simulink model "fwv_modified"  (R2021b)
settings: Solver=ode15s  StartTime=0.0  StopTime=10  FixedStep=0.01  MaxStep=0.01  RelTol=1e-3  AbsTol=1e-3  EnableMultiTasking=on
model workspace (MATLAB code in the model file):
  | p0=[0 0 0];
undefined symbols (not defined in the file): A_D, A_L, adpk, adps, c_bar, C_D0, il, ol, psi0, r00, r11, r22, r33, r_cp, rho, Rw, X, Y, Z, z00, z11, z22, zrd
libraries: sm_lib x54, nesl_utility x45, vrlib x3
(part 1 of 3)
settings Model: NumberOfSteps=10  PacingRate=1000  Creator=jeff  LastModifiedBy=jeff
settings SolverCC: AutoScaleAbsTol=off  ZeroCrossAlgorithm=Adaptive  SolverResetMethod=Robust
settings DataIOCC: LimitDataPoints=on  MaxDataPoints=10000  SignalLogging=off  DSMLogging=off  InspectSignalLogs=on  SaveTime=off  ReturnWorkspaceOutputs=off
settings OptimizationCC: LifeSpan=inf
settings DebuggingCC: AllowSymbolicDim=off  SFUnexpectedBacktrackingDiag=warning  SFNoUnconditionalDefaultTransitionDiag=warning  SFExecutionAtInitializationDiag=none  SFMachineParentedDataDiag=warning  ArithmeticOperatorsInVariantConditions=warning
settings ModelReferenceCC: ModelReferenceMinAlgLoopOccurrences=on
settings SFSimCC: SimUseLocalCustomCode=off  CustomCodeUndefinedFunction=UseInterfaceOnly
settings RTWCC: RTWUseLocalCustomCode=off
settings CodeAppCC: StateflowObjectComments=on
settings GRTTargetCC: TargetLangStandard=C89/C90 (ANSI)
settings ConfigComp: CovMetricSettings=dw  CovSaveCumulativeToWorkspaceVar=on  CovSaveSingleToWorkspaceVar=on  CovExternalEMLEnable=off  CovSFcnEnable=off
settings SimscapeCC: SimscapeLogType=all  SimscapeLogSimulationStatistics=on  SimscapeLogDataHistory=10000
settings ExplorerConfigSet: InternalSimMechanicsExplorerSettings="<ExplorerConfiguration><canonicalview>default</canonicalview><AnimationSetting><BasePlaybackSpeed>1.0</BasePlaybackSpeed><PlaybackSpeedFactor>1.0</PlaybackSpeedFactor></AnimationSetting><TilePanel><TileInfo><Tiles Columns=\"2\" Count=\"4\" Rows=\"2\"><Column Weight=\"0.5\"/><Column Weight=\"0.5\"/><Row Weight=\"0.4982\"/><Row Weight=\"0.5018\"/><Tile Height=\"1\" Width=\"1\" X=\"0\" Y=\"0\"/><Tile Height=\"1\" Width=\"1\" X=\"0\" Y=\"1\"/><Tile Height=\"1\" Width=\"1\" X=\"1\" Y=\"0\"/><Tile Height=\"1\" Width=\"1\" X=\"1\" Y=\"1\"/></Tiles></TileInfo><SceneInfo><SceneViewer><BGColor><R>1</R><G>1</G><B>1</B></BGColor><Camera><DoPerspective>off</DoPerspective><Position><X>0.641396731553975696</X><Y>-14.1815569735496414</Y><Z>0.672169191527196008</Z></Position><Center><X>0.641396731553975696</X><Y>-2.76871848114979002e-07</Y><Z>0.672169191527196008</Z></Center><Up><X>0</X><Y>-0</Y><Z>1</Z></Up><ViewLimDist>1</ViewLimDist><YLim>0.799989355072956321</YLim><XLim>1.08260667709303204</XLim></Camera></SceneViewer><SceneViewer><BGColor><R>1</R><G>1</G><B>1</B></BGColor><Camera><DoPerspective>off</DoPerspective><Position><X>-0.159012287126067881</X><Y>0.579024453304961995</Y><Z>14.2124818348279263</Z></Position><Center><X>-0.159012287126067881</X><Y>0.579024453304961995</Y><Z>-0.00300049176476058221</Z></Center><Up><X>0</X><Y>1</Y><Z>-0</Z></Up><ViewLimDist>1</ViewLimDist><YLim>3.05791516459476309</YLim><XLim>4.10313475475286005</XLim></Camera></SceneViewer><SceneViewer><BGColor><R>1</R><G>1</G><B>1</B></BGColor><Camera><DoPerspective>off</DoPerspective><Position><X>14.1815569760706541</X><Y>0.198096922096877126</Y><Z>0.664029497099502652</Z></Position><Center><X>-9.47977211396278108e-07</X><Y>0.198096922096877126</Y><Z>0.664029497099502652</Z></Center><Up><X>-0</X><Y>0</Y><Z>1</Z></Up><ViewLimDist>1</ViewLimDist><YLim>0.784069566907004467</YLim><XLim>1.06106280421888055</XLim></Camera></SceneViewer><SceneViewer><BGColor><R>1</R><G>1</G><B>1</B></BGColor><Camera><DoPerspective>on</DoPerspective><Position><X>0.900649549639901181</X><Y>0.398934934644883776</Y><Z>0.90015424109364861</Z></Position><Center><X>0.500649549639901048</X><Y>0.398934934644883721</Y><Z>0.800154241093648633</Z></Center><Up><X>0</X><Y>-3.08148791101957736e-33</Y><Z>1</Z></Up><ViewLimDist>1</ViewLimDist><YLim>0.466307658154998583</YLim><XLim>0.625695304021537613</XLim></Camera></SceneViewer></SceneInfo></TilePanel><MechEditorPanel><Cameras><Camera><Id>Camera1</Id><Value><Name>Camera1</Name><NativeCamera><PositionTrackingFeature>FWV.Body.camera.camera_Frame.R</PositionTrackingFeature><CenterTrackingFeature>FWV.Body.camera.C</CenterTrackingFeature><UpVectorTrackingFeature>FWV.Body.camera.C</UpVectorTrackingFeature><CenterTrackingOrigin>on</CenterTrackingOrigin><UpVectorTrackingDirection>+Z</UpVectorTrackingDirection></NativeCamera></Value></Camera></Cameras><GfxPanelCameraMap><MapElement CameraMLId=\"Camera1\" GfxPanelIndex=\"3\"/></GfxPanelCameraMap><VideoCreator><PlaybackSpeedRatio>1.0</PlaybackSpeedRatio><FrameRate>30</FrameRate><VideoFormat>Motion JPEG AVI</VideoFormat><FrameSize>[1280 720]</FrameSize></VideoCreator></MechEditorPanel></ExplorerConfiguration>"

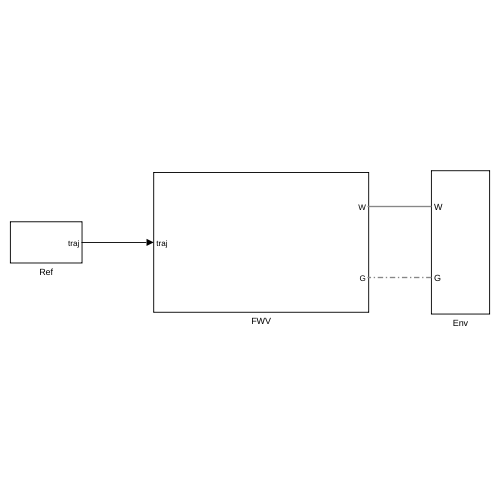
[thumbnail: Simulink's stored preview of the top-level diagram]
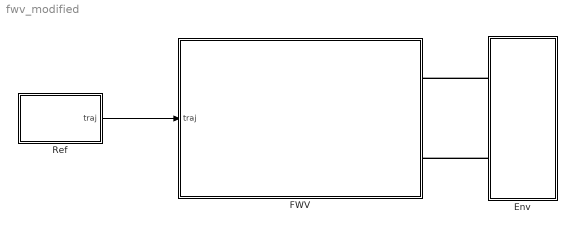
== system fwv_modified ==
  Env : Subsystem
  FWV : Subsystem
  Ref : Subsystem
  wires:
  Ref/1(traj) -> FWV/1(traj)
  connections:
  Env/LConn1 -- FWV/RConn1
  Env/LConn2 -- FWV/RConn2

== system fwv_modified/Env ==
  Ground : Subsystem
  Mechanism Configuration : sm_lib/Utilities/Mechanism Configuration  UniformGravity=Constant  GravityVector=[0 0 -9.80665]  GravityUnits=m/s^2  LinearizationDelta=0.001  JointModeTransitionNonlinearIterations=2
  Solver Configuration : nesl_utility/Solver Configuration  PhysicalDomain=network_engine_domain  SubClassName=solver  LeftPortType=input  RightPortType=generic  Tones=[]  Harmonics=[]  SimulateNoise=off  Profile=off  UseLocalSampling=off  EnableSwitchedLinearOptims=on  FrequencyDomain=off  UseCCode=off  RelTol=0.001  AbsTol=1e-06  MinStep=1e-09  ToWorkspace=off  RevertToSquareIcSolve=off  NumHomotopyIterations=100  PhasorMode=off  PhasorModeNumHarmonics=1  DoDC=off  ResidualTolerance=1e-09  UseLocalSolver=off  LocalSolverChoice=NE_BACKWARD_EULER_ADVANCER  LocalSolverSampleTime=0.001  DoFixedCost=off  MaxNonlinIter=3  MaxModeIter=2  ComputeImpulses=off  ImpulseIterations=2  LinearAlgebra=Sparse  EquationFormulation=NE_TIME_EF  DelaysMemoryBudget=1024  AutomaticFiltering=on  FilteringTimeConstant=0.001  PartitionStorageMethod=AS_NEEDED  PartitionMemoryBudget=1024  PartitionMethod=FAST
      settings: SourceProductBaseCode=PW,SS
  World Frame1 : sm_lib/Frames and Transforms/World Frame
  W : PMIOPort  Side=Left
  G : PMIOPort  Port=2  Side=Left
  connections:
  Ground/RConn1 -- G/RConn1
  Ground/LConn1 -- Mechanism Configuration/RConn1 -- World Frame1/RConn1 -- Solver Configuration/RConn1 -- W/RConn1

== system fwv_modified/FWV ==
  traj : Inport
  Body : Subsystem  mask{rho_w=900, m_t=20, stif_stk=0, stif_rot=5e-2, damp_rot=0, stif_m=1e2, damp_m=1e2, p0=p0, phi0=0, theta0=0, psi0=psi0}
      mask prompts: p0 "initial position(m)"; phi0 "initial roll(rad)"; theta0 "initial pitch(rad)"; psi0 "initial yaw(rad)"
      mask Display: image('Images/fwv.png');
  Controller : Subsystem
  Visualization : Subsystem
  W : PMIOPort  Side=Right
  G : PMIOPort  Port=2  Side=Right
  wires:
  Controller/1(ctrl) -> Body/1(ctrl)
  Body/1(state) -> Visualization/1(state), Controller/1(state)
  traj/1 -> Visualization/2(traj), Controller/2(Traj)
  connections:
  W/RConn1 -- Body/LConn1
  G/RConn1 -- Body/RConn1

== system fwv_modified/Ref ==
  Clock : Clock
  Mux : Mux  Inputs=6
  To Workspace : ToWorkspace  VariableName=t  SampleTime=-1
  p,pdot,pddot : MATLAB Function  TreatAsAtomicUnit=on
  traj : Outport
  wires:
  Mux/1 -> traj/1
  p,pdot,pddot/1(p) -> Mux/1  "p"
  p,pdot,pddot/2(heading) -> Mux/2
  p,pdot,pddot/3(v) -> Mux/3  "v"
  p,pdot,pddot/4(heading_dot) -> Mux/4
  p,pdot,pddot/5(a) -> Mux/5  "a"
  p,pdot,pddot/6(heading_ddot) -> Mux/6
  Clock/1 -> To Workspace/1, p,pdot,pddot/1(t)

== system fwv_modified/Env/Ground ==
  Cylindrical Solid : sm_lib/Body Elements/Cylindrical Solid  GraphicAmbientColor=[0.15 0.15 0.15 1.0]  BasedOnType=Mass  CenterOfMass=[0 0 0]  CenterOfMassUnits=m  GraphicDiffuseColor=[0.8 1.0 0.8]  CylinderLength=10  CylinderLengthUnits=mm  CylinderRadius=4  CylinderRadiusUnits=m  Density=1000  DensityUnits=kg/m^3  DoExposeReferenceFrame=off  GraphicEmissiveColor=[0.0 0.0 0.0 1.0]  ExportEntireGeometry=on  SerializedFrames=<Frames><Frame><Id>Frame1</Id><Value><Name>F1</Name><Origin><Source>GeometricFeature</Source><FeatureName>top surface</FeatureName></Origin><PrimaryAxis><DefinedDirection>+Z</DefinedDirection><Source>ReferenceFrame</Source><SourceDirection>+Z</SourceDirection><FeatureName></FeatureName></PrimaryAxis><SecondaryAxis><DefinedDirection>+X</DefinedDirection><Source>ReferenceFrame</Source><SourceDirection>+X</SourceDirection><FeatureName></FeatureName></SecondaryAxis></Value></Frame></Frames>  MarkerShape=Sphere  MarkerSize=10  GraphicType=FromGeometry  InertiaType=Custom  Mass=0  MassUnits=kg  MomentsOfInertia=[1 1 1]  MomentsOfInertiaUnits=kg*m^2  GraphicOpacity=1.0  ProductsOfInertia=[0 0 0]  ProductsOfInertiaUnits=kg*m^2  GraphicShininess=75  GraphicSpecularColor=[0.5 0.5 0.5 1.0]  GraphicVisPropType=SimpleVisualProperties
  Rigid Transform : sm_lib/Frames and Transforms/Rigid Transform  TranslationMethod=StandardAxis  TranslationStandardOffset=6  TranslationLengthUnit=cm  TranslationStandardAxis=-Z  TranslationCartesianOffset=[0 0 0]  TranslationROffset=0  TranslationROffsetUnits=m  TranslationZOffset=0  TranslationZOffsetUnits=m  TranslationThetaOffset=0  TranslationThetaOffsetUnits=deg  RotationMethod=None  RotationAngleUnits=deg  RotationStandardAxis=+Z  RotationAngle=0.0  RotationArbitraryAxis=[0 0 1]  FollAlignAxisA=+X  BaseAlignAxisA=+Y  FollAlignAxisB=+Y  BaseAlignAxisB=+Z  RotationSequenceAxes=FollowerAxes  RotationSequence=XYX  RotationSequenceAngles=[0 0 0]  RotationSequenceAnglesUnits=deg  RotationMatrix=[1 0 0; 0 1 0; 0 0 1]
  W : PMIOPort  Side=Left
  G : PMIOPort  Port=2  Side=Right
  connections:
  G/RConn1 -- Cylindrical Solid/RConn1
  Rigid Transform/LConn1 -- W/RConn1
  Rigid Transform/RConn1 -- Cylindrical Solid/LConn1

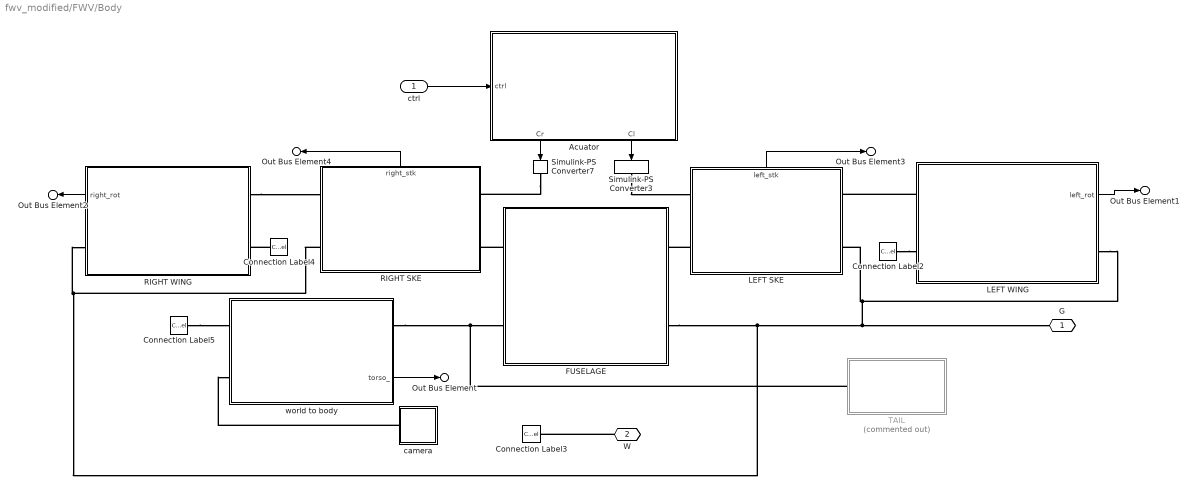
== system fwv_modified/FWV/Body ==
  ctrl : Inport
  Acuator : Subsystem
      settings: PortSchema="{\"entries\":[{\"content\":{\"sides\":[{\"content\":{\"connectorIds\":[\"In1\"]},\"type\":\"ConnectorPlacement.EquallySpacedRectSide\",\"uuid\":\"db46f0ff-2b35-4735-b2ba-99ebad500531\"},{\"content\":{\"connectorIds\":[],\"side\":\"RIGHT\"},\"type\":\"ConnectorPlacement.EquallySpacedRectSide\",\"uuid\":\"a05d2a9d-5b8e-445a-bb52-abca9ea78047\"},{\"content\":{\"connectorIds\":[],\"side\":\"TOP\"},\"type\":\"ConnectorPlacement.EquallySpacedRectSide\",\"uuid\":\"a9e07a0b-59af-45c6-89e8-be07490c71bb\"},{\"content\":{\"connectorIds\":[\"Out1\",\"Out2\"],\"side\":\"BOTTOM\"},\"type\":\"ConnectorPlacement.EquallySpacedRectSide\",\"uuid\":\"69a70806-995a-45b1-874e-667630f2a15c\"}]},\"type\":\"ConnectorPlacement.EquallySpacedConnector\",\"uuid\":\"cc8e5811-56fa-45cd-8c97-474062c30ea3\"}],\"packageUris\":[\"http://schema.mathworks.com/mf0/Connector/R2020b\"],\"version\":\"1.0\"}"
  Connection Label{2..5} (4 alike) : ConnectionLabel  Label=W
  FUSELAGE : Subsystem  mask{mu0=0, mu1=0}
      mask Display: image('Images/fuselage.png'); % Use "Edit Image" on toolstrip to change.
  LEFT SKE : Subsystem
      settings: PortSchema="{\"entries\":[{\"content\":{\"sides\":[{\"content\":{\"connectorIds\":[\"LConn1\",\"LConn2\"]},\"type\":\"ConnectorPlacement.EquallySpacedRectSide\",\"uuid\":\"e449d641-3a3a-4b99-9659-b7cfb3580d3e\"},{\"content\":{\"connectorIds\":[\"RConn1\",\"RConn2\"],\"side\":\"RIGHT\"},\"type\":\"ConnectorPlacement.EquallySpacedRectSide\",\"uuid\":\"c0f0c2d4-a937-4da0-b288-84b9bdeda0ec\"},{\"content\":{\"connectorIds\":[\"Out1\"],\"side\":\"TOP\"},\"type\":\"ConnectorPlacement.EquallySpacedRectSide\",\"uuid\":\"2e9a5fca-fc91-474a-9824-391ef1d64046\"}]},\"type\":\"ConnectorPlacement.EquallySpacedConnector\",\"uuid\":\"1b8d15a7-e855-4706-95be-75cb969fd455\"}],\"packageUris\":[\"http://schema.mathworks.com/mf0/Connector/R2020b\"],\"version\":\"1.0\"}"
      mask Display: image('Images/lle.png'); % Use "Edit Image" on toolstrip to change.
  LEFT WING : Subsystem
      mask Display: image('Images/lwing.png'); % Use "Edit Image" on toolstrip to change.
  RIGHT SKE : Subsystem
      settings: PortSchema="{\"entries\":[{\"content\":{\"sides\":[{\"content\":{\"connectorIds\":[\"LConn1\",\"LConn2\"]},\"type\":\"ConnectorPlacement.EquallySpacedRectSide\",\"uuid\":\"e80f0529-82a8-4e91-8f70-1f5fff48efb0\"},{\"content\":{\"connectorIds\":[\"RConn1\",\"RConn2\"],\"side\":\"RIGHT\"},\"type\":\"ConnectorPlacement.EquallySpacedRectSide\",\"uuid\":\"c7e3ee7d-7bee-46da-b210-768e5832b89d\"},{\"content\":{\"connectorIds\":[\"Out1\"],\"side\":\"TOP\"},\"type\":\"ConnectorPlacement.EquallySpacedRectSide\",\"uuid\":\"680cbd67-40e5-4a58-a196-f2062cf587c7\"}]},\"type\":\"ConnectorPlacement.EquallySpacedConnector\",\"uuid\":\"7cb1a5ec-7352-40bf-9e6c-a29cba360f94\"}],\"packageUris\":[\"http://schema.mathworks.com/mf0/Connector/R2020b\"],\"version\":\"1.0\"}"
      mask Display: image('Images/rle.png'); % Use "Edit Image" on toolstrip to change.
  RIGHT WING : Subsystem
      mask Display: image('Images/rwing.png'); % Use "Edit Image" on toolstrip to change.
  Simulink-PS Converter3 : nesl_utility/Simulink-PS Converter  PhysicalDomain=network_engine_domain  SubClassName=ps_input  LeftPortType=input  RightPortType=output  PseudoPeriodic=off  Frequencies=[]  NoiseDistribution=none  NoiseParameters=[]  Unit=1  AffineConversion=off  FilteringAndDerivatives=filter  SimscapeFilterOrder=2  InputFilterTimeConstant=0.001  UdotUserProvided=2
      settings: SourceProductBaseCode=PW,SS
  Simulink-PS Converter7 : nesl_utility/Simulink-PS Converter  PhysicalDomain=network_engine_domain  SubClassName=ps_input  LeftPortType=input  RightPortType=output  PseudoPeriodic=off  Frequencies=[]  NoiseDistribution=none  NoiseParameters=[]  Unit=1  AffineConversion=off  FilteringAndDerivatives=filter  SimscapeFilterOrder=2  InputFilterTimeConstant=0.001  UdotUserProvided=0
      settings: SourceProductBaseCode=PW,SS
  TAIL : Subsystem  Commented=on
  camera : Subsystem
  world to body : Subsystem
      settings: PortSchema="{\"entries\":[{\"content\":{\"sides\":[{\"content\":{\"connectorIds\":[\"LConn1\",\"LConn2\"]},\"type\":\"ConnectorPlacement.EquallySpacedRectSide\",\"uuid\":\"67e08b7d-27a7-478e-aa2b-0a29cfb8c4ba\"},{\"content\":{\"connectorIds\":[\"RConn1\",\"Out1\"],\"side\":\"RIGHT\"},\"type\":\"ConnectorPlacement.EquallySpacedRectSide\",\"uuid\":\"af848fd7-c404-4734-a34f-7cffff1411b1\"},{\"content\":{\"connectorIds\":[],\"side\":\"TOP\"},\"type\":\"ConnectorPlacement.EquallySpacedRectSide\",\"uuid\":\"40c86437-2469-4d2e-8b61-7b3eee85e893\"}]},\"type\":\"ConnectorPlacement.EquallySpacedConnector\",\"uuid\":\"cd10b607-3f85-4cd2-a6c3-0d07bf2597bd\"}],\"packageUris\":[\"http://schema.mathworks.com/mf0/Connector/R2020b\"],\"version\":\"1.0\"}"
  G : PMIOPort  Side=Right
  W : PMIOPort  Port=2  Side=Left
  Out Bus Element : Outport  PortName=state  Element=pose
  Out Bus Element3 : Outport  PortName=state  Element=left_stk
  Out Bus Element1 : Outport  PortName=state  Element=left_rot
  Out Bus Element4 : Outport  PortName=state  Element=right_stk
  Out Bus Element2 : Outport  PortName=state  Element=right_rot
  wires:
  LEFT WING/1(left_rot) -> Out Bus Element1/1
  RIGHT WING/1(right_rot) -> Out Bus Element2/1
  world to body/1(torso_) -> Out Bus Element/1
  Acuator/2(Cl) -> Simulink-PS Converter3/1
  Acuator/1(Cr) -> Simulink-PS Converter7/1
  ctrl/1 -> Acuator/1(ctrl)
  LEFT SKE/1(left_stk) -> Out Bus Element3/1
  RIGHT SKE/1(right_stk) -> Out Bus Element4/1
  connections:
  LEFT SKE/LConn2 -- FUSELAGE/RConn1
  FUSELAGE/LConn1 -- RIGHT SKE/RConn2
  Simulink-PS Converter7/RConn1 -- RIGHT SKE/RConn1
  world to body/RConn1 -- TAIL/LConn1 -- FUSELAGE/LConn2
  camera/LConn1 -- world to body/LConn2
  Simulink-PS Converter3/RConn1 -- LEFT SKE/LConn1
  LEFT WING/LConn1 -- LEFT SKE/RConn1
  RIGHT WING/LConn1 -- RIGHT SKE/LConn1
  Connection Label2/LConn1 -- LEFT WING/LConn2
  Connection Label4/LConn1 -- RIGHT WING/LConn2
  Connection Label5/LConn1 -- world to body/LConn1
  W/RConn1 -- Connection Label3/LConn1
  RIGHT SKE/LConn2 -- G/RConn1 -- LEFT SKE/RConn2 -- LEFT WING/RConn1 -- FUSELAGE/RConn2 -- RIGHT WING/RConn1

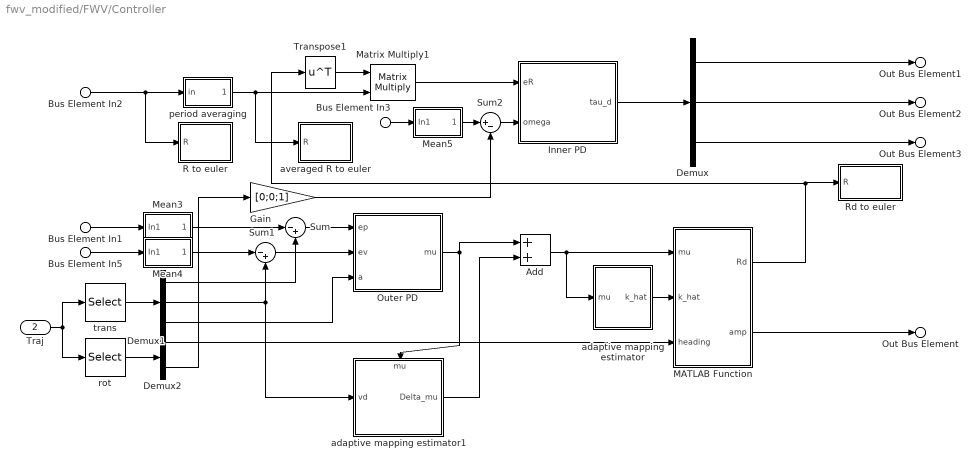
== system fwv_modified/FWV/Controller ==
  Bus Element In1 : Inport  PortName=state  Element=pose.p
  Bus Element In2 : Inport  PortName=state  Element=pose.R
  Bus Element In3 : Inport  PortName=state  Element=pose.w
  Bus Element In5 : Inport  PortName=state  Element=pose.v
  Traj : Inport  Port=2
  Add : Sum
  Demux : Demux  Outputs=3
  Demux1 : Demux  Outputs=3
  Demux2 : Demux  Outputs=2
  Gain : Gain  Gain=[0;0;1]
  Inner PD : Subsystem
  MATLAB Function : MATLAB Function  TreatAsAtomicUnit=on
  Matrix Multiply1 : Product  Multiplication=Matrix(*)
  Mean3 : Subsystem
  Mean4 : Subsystem
  Mean5 : Subsystem
  Outer PD : Subsystem
  R to euler : Subsystem
  Rd to euler : Subsystem
      settings: PortSchema="{\"entries\":[{\"content\":{\"sides\":[{\"content\":{\"connectorIds\":[]},\"type\":\"ConnectorPlacement.EquallySpacedRectSide\",\"uuid\":\"93de112d-0217-40d7-a336-17ea7cc4ed84\"},{\"content\":{\"connectorIds\":[\"In1\"],\"side\":\"RIGHT\"},\"type\":\"ConnectorPlacement.EquallySpacedRectSide\",\"uuid\":\"0b203bc8-f5c1-4f94-b862-0e0b0c3261f7\"},{\"content\":{\"connectorIds\":[],\"side\":\"TOP\"},\"type\":\"ConnectorPlacement.EquallySpacedRectSide\",\"uuid\":\"1be19d4c-6517-470f-aabd-96bb4bcaed3d\"}]},\"type\":\"ConnectorPlacement.EquallySpacedConnector\",\"uuid\":\"f5fc68b0-193c-43e6-a8c2-776496b24de9\"}],\"packageUris\":[\"http://schema.mathworks.com/mf0/Connector/R2020b\"],\"version\":\"1.0\"}"
  Sum : Sum  Inputs=|-+
  Sum1 : Sum  Inputs=|-+
  Sum2 : Sum  Inputs=|+-
  Transpose1 : Math  Operator=transpose  SaturateOnIntegerOverflow=on
  adaptive mapping estimator : Subsystem
  adaptive mapping estimator1 : Subsystem
      settings: PortSchema="{\"entries\":[{\"content\":{\"sides\":[{\"content\":{\"connectorIds\":[\"In1\"]},\"type\":\"ConnectorPlacement.EquallySpacedRectSide\",\"uuid\":\"ad990f9c-fb26-46a0-b20f-9b75f9cabb9c\"},{\"content\":{\"connectorIds\":[\"Out1\"],\"side\":\"RIGHT\"},\"type\":\"ConnectorPlacement.EquallySpacedRectSide\",\"uuid\":\"f73f0012-14a6-4c3b-b3ee-1c6141b5dee9\"},{\"content\":{\"connectorIds\":[\"In2\"],\"side\":\"TOP\"},\"type\":\"ConnectorPlacement.EquallySpacedRectSide\",\"uuid\":\"988c0ea2-b49a-4053-a70e-8b43fa663825\"}]},\"type\":\"ConnectorPlacement.EquallySpacedConnector\",\"uuid\":\"beeb5652-2bef-4034-a2ae-37ff7c082bb3\"}],\"packageUris\":[\"http://schema.mathworks.com/mf0/Connector/R2020b\"],\"version\":\"1.0\"}"
  averaged R to euler : Subsystem
  period averaging : Subsystem
  rot : Selector  InputPortWidth=12  IndexOptions=Index vector (dialog)  Indices=[4 8]  OutputSizes=1
  trans : Selector  InputPortWidth=12  IndexOptions=Index vector (dialog)  Indices=[1 2 3 5 6 7 9 10 11]  OutputSizes=1
  Out Bus Element : Outport  PortName=ctrl  Element=amp_mean
  Out Bus Element1 : Outport  PortName=ctrl  Element=amp_diff
  Out Bus Element2 : Outport  PortName=ctrl  Element=bias
  Out Bus Element3 : Outport  PortName=ctrl  Element=offset
  wires:
  Demux1/1 -> Sum/2
  Inner PD/1(tau_d) -> Demux/1
  Transpose1/1 -> Matrix Multiply1/1
  Demux1/2 -> adaptive mapping estimator1/1(vd), Sum1/2
  Demux1/3 -> Outer PD/3(a)
  Bus Element In2/1 -> R to euler/1(R), period averaging/1(in)
  Demux2/1 -> MATLAB Function/3(heading)
  Sum/1 -> Outer PD/1(ep)
  Sum1/1 -> Outer PD/2(ev)
  Matrix Multiply1/1 -> Inner PD/1(eR)
  MATLAB Function/1(Rd) -> Transpose1/1, Rd to euler/1(R)
  Bus Element In1/1 -> Mean3/1(In1)
  Bus Element In5/1 -> Mean4/1(In1)
  Mean3/1(Mean1) -> Sum/1
  Mean4/1(Mean1) -> Sum1/1
  Bus Element In3/1 -> Mean5/1(In1)
  MATLAB Function/2(amp) -> Out Bus Element/1
  period averaging/1(Mean1) -> averaged R to euler/1(R), Matrix Multiply1/2
  adaptive mapping estimator/1(k_hat) -> MATLAB Function/2(k_hat)
  Demux/1 -> Out Bus Element1/1
  Demux/2 -> Out Bus Element2/1
  Demux/3 -> Out Bus Element3/1
  Mean5/1(Mean1) -> Sum2/1
  Sum2/1 -> Inner PD/2(omega)
  Demux2/2 -> Gain/1
  Gain/1 -> Sum2/2
  trans/1 -> Demux1/1
  rot/1 -> Demux2/1
  Traj/1 -> rot/1, trans/1
  adaptive mapping estimator1/1(Delta_mu) -> Add/2
  Add/1 -> adaptive mapping estimator/1(mu), MATLAB Function/1(mu)
  Outer PD/1(mu) -> adaptive mapping estimator1/2(mu), Add/1

== system fwv_modified/FWV/Visualization ==
  Bus Element In1 : Inport  PortName=state  Element=pose.p
  Bus Element In2 : Inport  PortName=state  Element=pose.R
  traj : Inport  Port=2
  Demux : Demux  Outputs=3
  Mux : Mux  Inputs=2
  Selector : Selector  InputPortWidth=12  IndexOptions=Index vector (dialog)  Indices=[1 2 3 4]  OutputSizes=1
  Subsystem : Subsystem
  Terminator : Terminator
  To Workspace : ToWorkspace  VariableName=q  SampleTime=-1
      settings: Save2DSignal=2-D array (concatenate along first dimension)
  To Workspace1 : ToWorkspace  VariableName=qd  SampleTime=-1
      settings: Save2DSignal=2-D array (concatenate along first dimension)
  XY Graph : Record  FileSettingsInternal="{\"entries\":[{\"content\":{\"excelSettings\":{\"content\":{},\"type\":\"Streamout.ExcelSettings\"}},\"type\":\"Streamout.FileSettingStorage\",\"uuid\":\"9068cc09-93f0-4c38-80ae-0346da1374ca\"}],\"packageUris\":[\"http://schema.mathworks.com/mf0/streamout_blocks/R2020a\"],\"version\":\"1.0\"}"  Layout=[1 1]  SignalsInternal="{\"entries\":[{\"content\":{\"signals\":[{\"content\":{\"blockPath\":[\"fwv_modified/FWV/Visualization/XY Graph\"],\"channel\":[],\"dimensions\":[1],\"domain\":\"fwv_modified/FWV/Visualization/XY Graph\",\"lineColor\":\"#139fff\",\"plots\":[],\"port\":1,\"sid\":[],\"signalID\":199,\"signalName\":\"Demux:1\"},\"type\":\"RecordBlkView.Signal\",\"uuid\":\"b9a14841-9106-4e77-be14-2ac67169168d\"},{\"content\":{\"blockPath\":[\"fwv_modified/FWV/Visualization/XY Graph\"],\"channel\":[],\"dimensions\":[1],\"domain\":\"fwv_modified/FWV/Visualization/XY Graph\",\"lineColor\":\"#ff6929\",\"plots\":[],\"port\":2,\"sid\":[],\"signalID\":202,\"signalName\":\"Demux:2\"},\"type\":\"RecordBlkView.Signal\",\"uuid\":\"9ba150dd-5ced-4f31-a10c-923c26d79fdc\"}]},\"type\":\"RecordBlkView.InputSignals\",\"uuid\":\"991fd4fc-8561-4340-9e61-2b96f507fad7\"}],\"packageUris\":[\"http://schema.mathworks.com/mf0/streamout_blocks/R2020a\"],\"version\":\"1.0\"}"  VisualizationBindings="{\"xyplotplugin\":{\"info\":[{\"series\":[],\"subplotID\":1}]}}"  CompatibilityTag=XY  st=-1
  wires:
  Bus Element In1/1 -> Mux/1, Demux/1
  Demux/3 -> Terminator/1
  Demux/1 -> XY Graph/1
  Demux/2 -> XY Graph/2
  Selector/1 -> To Workspace1/1
  traj/1 -> Selector/1
  Bus Element In2/1 -> Subsystem/1(R)
  Subsystem/1(yaw) -> Mux/2
  Mux/1 -> To Workspace/1

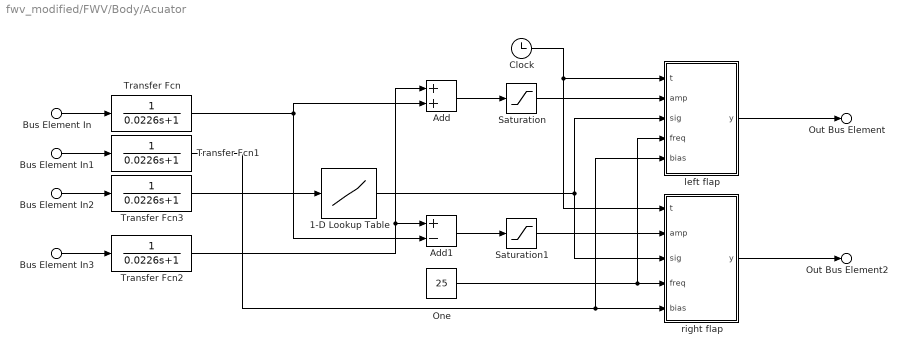
== system fwv_modified/FWV/Body/Acuator ==
  Bus Element In3 : Inport  PortName=ctrl  Element=amp_mean
  Bus Element In : Inport  PortName=ctrl  Element=amp_diff
  Bus Element In1 : Inport  PortName=ctrl  Element=bias
  Bus Element In2 : Inport  PortName=ctrl  Element=offset
  " left flap" : MATLAB Function  TreatAsAtomicUnit=on
  " right flap" : MATLAB Function  TreatAsAtomicUnit=on
  1-D Lookup Table : Lookup_n-D  NumberOfTableDimensions=1  BreakpointsForDimension1=[-1:1]  Table=1.0./(1+exp(-10*[-1:1]))  InternalRulePriority=Speed  RndMeth=Simplest  InputSameDT=on
  Add : Sum
  Add1 : Sum  Inputs=+-
  Clock : Clock
  One : Constant  Value=25  OutDataTypeStr=Inherit: Inherit via back propagation
  Saturation : Saturate  UpperLimit=pi/2  LowerLimit=0  ZeroCross=off
  Saturation1 : Saturate  UpperLimit=pi/2  LowerLimit=0  ZeroCross=off
  Transfer Fcn{,1..3} (4 alike) : TransferFcn  Denominator=[0.0226 1]
  Out Bus Element2 : Outport  PortName=Cr  Element=stroke
  Out Bus Element : Outport  Port=2  PortName=Cl  Element=stroke
  wires:
  Add1/1 -> Saturation1/1
  " left flap"/1(y) -> Out Bus Element/1
  One/1 -> " left flap"/4(freq), " right flap"/4(freq)
  " right flap"/1(y) -> Out Bus Element2/1
  Add/1 -> Saturation/1
  Saturation/1 -> " left flap"/2(amp)
  Clock/1 -> " right flap"/1(t), " left flap"/1(t)
  Saturation1/1 -> " right flap"/2(amp)
  Transfer Fcn2/1 -> Add/1, Add1/1
  Transfer Fcn/1 -> Add1/2, Add/2
  Bus Element In/1 -> Transfer Fcn/1
  Bus Element In1/1 -> Transfer Fcn1/1
  Bus Element In2/1 -> Transfer Fcn3/1
  Bus Element In3/1 -> Transfer Fcn2/1
  Transfer Fcn1/1 -> " left flap"/5(bias), " right flap"/5(bias)
  Transfer Fcn3/1 -> 1-D Lookup Table/1
  1-D Lookup Table/1 -> " right flap"/3(sig), " left flap"/3(sig)

== system fwv_modified/FWV/Body/FUSELAGE ==
  note: Contact Measurement
  Rigid Transform : sm_lib/Frames and Transforms/Rigid Transform  TranslationMethod=StandardAxis  TranslationStandardOffset=5.75  TranslationLengthUnit=cm  TranslationStandardAxis=-Z  TranslationCartesianOffset=[0 0 0]  TranslationROffset=0  TranslationROffsetUnits=m  TranslationZOffset=0  TranslationZOffsetUnits=m  TranslationThetaOffset=0  TranslationThetaOffsetUnits=deg  RotationMethod=RotationSequence  RotationAngleUnits=deg  RotationStandardAxis=+Y  RotationAngle=90  RotationArbitraryAxis=[0 0 1]  FollAlignAxisA=+X  BaseAlignAxisA=+Y  FollAlignAxisB=+Y  BaseAlignAxisB=+Z  RotationSequenceAxes=FollowerAxes  RotationSequence=ZYX  RotationSequenceAngles=[45 90 0]  RotationSequenceAnglesUnits=deg  RotationMatrix=[1 0 0; 0 1 0; 0 0 1]
  Rigid Transform1 : sm_lib/Frames and Transforms/Rigid Transform  TranslationMethod=StandardAxis  TranslationStandardOffset=5.75  TranslationLengthUnit=cm  TranslationStandardAxis=-Z  TranslationCartesianOffset=[0 0 0]  TranslationROffset=0  TranslationROffsetUnits=m  TranslationZOffset=0  TranslationZOffsetUnits=m  TranslationThetaOffset=0  TranslationThetaOffsetUnits=deg  RotationMethod=RotationSequence  RotationAngleUnits=deg  RotationStandardAxis=+X  RotationAngle=90  RotationArbitraryAxis=[0 0 1]  FollAlignAxisA=+X  BaseAlignAxisA=+Y  FollAlignAxisB=+Y  BaseAlignAxisB=+Z  RotationSequenceAxes=FollowerAxes  RotationSequence=ZYX  RotationSequenceAngles=[-45 90 0]  RotationSequenceAnglesUnits=deg  RotationMatrix=[1 0 0; 0 1 0; 0 0 1]
  Spatial Contact Force : sm_lib/Forces and Torques/Spatial Contact Force  CoefficientOfDynamicFriction=0.3  CoefficientOfStaticFriction=0.5  SenseContactBaseRotation=off  SenseContactBaseTranslation=off  NormalDamping=1e3  NormalDampingUnits=N/(m/s)  SenseContactFollowerRotation=off  SenseContactFollowerTranslation=off  SenseContactSignal=off  NormalStiffness=1e6  NormalStiffnessUnits=N/m  FrictionalCriticalVelocity=1e-3  FrictionalCriticalVelocityUnits=m/s  ZeroCrossDetectContactStartAndEnd=off  FrictionType=SmoothStickSlip  SenseFrictionalForceMagnitude=off  SenseNormalForceMagnitude=off  NormalForceType=SmoothSpringDamper  SenseNormalVelocity=off  SenseSeparationDistance=off  SenseTangentialVelocity=off  SenseTangentialVelocityMagnitude=off  NormalTransitionRegionWidth=1e-4  NormalTransitionRegionWidthUnits=m
  Spatial Contact Force1 : sm_lib/Forces and Torques/Spatial Contact Force  CoefficientOfDynamicFriction=0.3  CoefficientOfStaticFriction=0.5  SenseContactBaseRotation=off  SenseContactBaseTranslation=off  NormalDamping=1e3  NormalDampingUnits=N/(m/s)  SenseContactFollowerRotation=off  SenseContactFollowerTranslation=off  SenseContactSignal=off  NormalStiffness=1e6  NormalStiffnessUnits=N/m  FrictionalCriticalVelocity=1e-3  FrictionalCriticalVelocityUnits=m/s  ZeroCrossDetectContactStartAndEnd=off  FrictionType=SmoothStickSlip  SenseFrictionalForceMagnitude=off  SenseNormalForceMagnitude=off  NormalForceType=SmoothSpringDamper  SenseNormalVelocity=off  SenseSeparationDistance=off  SenseTangentialVelocity=off  SenseTangentialVelocityMagnitude=off  NormalTransitionRegionWidth=1e-4  NormalTransitionRegionWidthUnits=m
  Spatial Contact Force2 : sm_lib/Forces and Torques/Spatial Contact Force  CoefficientOfDynamicFriction=0.3  CoefficientOfStaticFriction=0.5  SenseContactBaseRotation=off  SenseContactBaseTranslation=off  NormalDamping=1e3  NormalDampingUnits=N/(m/s)  SenseContactFollowerRotation=off  SenseContactFollowerTranslation=off  SenseContactSignal=off  NormalStiffness=1e6  NormalStiffnessUnits=N/m  FrictionalCriticalVelocity=1e-3  FrictionalCriticalVelocityUnits=m/s  ZeroCrossDetectContactStartAndEnd=off  FrictionType=SmoothStickSlip  SenseFrictionalForceMagnitude=off  SenseNormalForceMagnitude=off  NormalForceType=SmoothSpringDamper  SenseNormalVelocity=off  SenseSeparationDistance=off  SenseTangentialVelocity=off  SenseTangentialVelocityMagnitude=off  NormalTransitionRegionWidth=1e-4  NormalTransitionRegionWidthUnits=m
  left_edge_of_torso : sm_lib/Frames and Transforms/Rigid Transform  TranslationMethod=Cartesian  TranslationStandardOffset=0  TranslationLengthUnit=cm  TranslationStandardAxis=+Z  TranslationCartesianOffset=[0 3.5 0]  TranslationROffset=0  TranslationROffsetUnits=m  TranslationZOffset=0  TranslationZOffsetUnits=m  TranslationThetaOffset=0  TranslationThetaOffsetUnits=deg  RotationMethod=None  RotationAngleUnits=deg  RotationStandardAxis=+Z  RotationAngle=0.0  RotationArbitraryAxis=[0 0 1]  FollAlignAxisA=+X  BaseAlignAxisA=+Y  FollAlignAxisB=+Y  BaseAlignAxisB=+Z  RotationSequenceAxes=FollowerAxes  RotationSequence=XYX  RotationSequenceAngles=[0 0 0]  RotationSequenceAnglesUnits=deg  RotationMatrix=[1 0 0; 0 1 0; 0 0 1]
  leg : sm_lib/Body Elements/Cylindrical Solid  GraphicAmbientColor=[0.15 0.15 0.15 1.0]  BasedOnType=Mass  CenterOfMass=[0 0 0]  CenterOfMassUnits=m  GraphicDiffuseColor=[0.5 0.5 0.5]  CylinderLength=160  CylinderLengthUnits=mm  CylinderRadius=2.5  CylinderRadiusUnits=mm  Density=1000  DensityUnits=kg/m^3  DoExposeReferenceFrame=on  GraphicEmissiveColor=[0.0 0.0 0.0 1.0]  ExportEntireGeometry=on  SerializedFrames=<Frames/>  MarkerShape=Sphere  MarkerSize=10  GraphicType=FromGeometry  InertiaType=CalculateFromGeometry  Mass=1  MassUnits=g  MomentsOfInertia=[1 1 1]  MomentsOfInertiaUnits=kg*m^2  GraphicOpacity=1.0  ProductsOfInertia=[0 0 0]  ProductsOfInertiaUnits=kg*m^2  GraphicShininess=75  GraphicSpecularColor=[0.5 0.5 0.5 1.0]  GraphicVisPropType=SimpleVisualProperties
  leg1 : sm_lib/Body Elements/Cylindrical Solid  GraphicAmbientColor=[0.15 0.15 0.15 1.0]  BasedOnType=Mass  CenterOfMass=[0 0 0]  CenterOfMassUnits=m  GraphicDiffuseColor=[0.5 0.5 0.5]  CylinderLength=160  CylinderLengthUnits=mm  CylinderRadius=2.5  CylinderRadiusUnits=mm  Density=800  DensityUnits=kg/m^3  DoExposeReferenceFrame=on  GraphicEmissiveColor=[0.0 0.0 0.0 1.0]  ExportEntireGeometry=on  SerializedFrames=<Frames/>  MarkerShape=Sphere  MarkerSize=10  GraphicType=FromGeometry  InertiaType=CalculateFromGeometry  Mass=1  MassUnits=g  MomentsOfInertia=[1 1 1]  MomentsOfInertiaUnits=kg*m^2  GraphicOpacity=1.0  ProductsOfInertia=[0 0 0]  ProductsOfInertiaUnits=kg*m^2  GraphicShininess=75  GraphicSpecularColor=[0.5 0.5 0.5 1.0]  GraphicVisPropType=SimpleVisualProperties
  right_edge_of_torso : sm_lib/Frames and Transforms/Rigid Transform  TranslationMethod=Cartesian  TranslationStandardOffset=0  TranslationLengthUnit=cm  TranslationStandardAxis=+Z  TranslationCartesianOffset=[0 -3.5 0]  TranslationROffset=0  TranslationROffsetUnits=m  TranslationZOffset=0  TranslationZOffsetUnits=m  TranslationThetaOffset=0  TranslationThetaOffsetUnits=deg  RotationMethod=StandardAxis  RotationAngleUnits=deg  RotationStandardAxis=+X  RotationAngle=180  RotationArbitraryAxis=[0 0 1]  FollAlignAxisA=+X  BaseAlignAxisA=+Y  FollAlignAxisB=+Y  BaseAlignAxisB=+Z  RotationSequenceAxes=FollowerAxes  RotationSequence=XYX  RotationSequenceAngles=[0 0 0]  RotationSequenceAnglesUnits=deg  RotationMatrix=[1 0 0; 0 1 0; 0 0 1]
  torso : sm_lib/Body Elements/File Solid  ExtGeomFileName=meshes/fuselage.stl  UnitType=Custom  ExtGeomFileUnits=mm  StepReaderType=HEX  ExportConvexHullGeometry=on  InertiaType=CalculateFromGeometry  Mass=m_t  MassUnits=g  CenterOfMass=[0 0 0]  CenterOfMassUnits=cm  MomentsOfInertia=[4e-5, 3e-5, 1.2e-5]  MomentsOfInertiaUnits=kg*m^2  ProductsOfInertia=[0 0 0]  ProductsOfInertiaUnits=kg*m^2  BasedOnType=Mass  Density=1000  DensityUnits=kg/m^3  DoExposeReferenceFrame=on  SerializedFrames=<Frames/>  GraphicType=FromGeometry  MarkerShape=Sphere  MarkerSize=10  GraphicVisPropType=SimpleVisualProperties  GraphicDiffuseColor=[0.5 0.5 0.5]  GraphicSpecularColor=[0.5 0.5 0.5 1.0]  GraphicAmbientColor=[0.15 0.15 0.15 1.0]  GraphicEmissiveColor=[0.0 0.0 0.0 1.0]  GraphicShininess=75  GraphicOpacity=1.0
  F1 : PMIOPort  Side=Right
  F2 : PMIOPort  Port=2  Side=Left
  TS : PMIOPort  Port=3  Side=Left
  G : PMIOPort  Port=4  Side=Right
  connections:
  Spatial Contact Force/RConn1 -- leg/LConn1
  Rigid Transform1/LConn1 -- torso/RConn1 -- right_edge_of_torso/LConn1 -- left_edge_of_torso/LConn1 -- Rigid Transform/LConn1 -- TS/RConn1
  Rigid Transform1/RConn1 -- leg1/RConn1
  left_edge_of_torso/RConn1 -- F1/RConn1
  leg/RConn1 -- Rigid Transform/RConn1
  F2/RConn1 -- right_edge_of_torso/RConn1
  Spatial Contact Force1/RConn1 -- leg1/LConn1
  G/RConn1 -- Spatial Contact Force2/LConn1 -- Spatial Contact Force1/LConn1 -- Spatial Contact Force/LConn1
  Spatial Contact Force2/RConn1 -- torso/LConn1

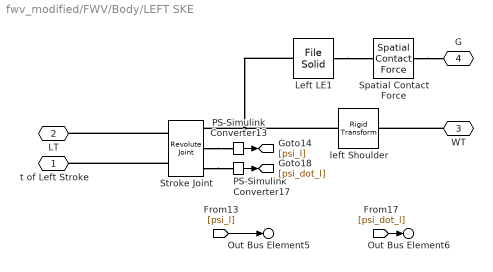
== system fwv_modified/FWV/Body/LEFT SKE ==
  Left LE1 : sm_lib/Body Elements/File Solid  ExtGeomFileName=meshes/left_LE.step  UnitType=FromFile  ExtGeomFileUnits=m  StepReaderType=HEX  ExportConvexHullGeometry=on  InertiaType=Custom  Mass=1  MassUnits=g  CenterOfMass=[0 0.0453 0.0239]  CenterOfMassUnits=m  MomentsOfInertia=[3.2e-06, 7.22e-07, 2.48e-06]  MomentsOfInertiaUnits=kg*m^2  ProductsOfInertia=[-7.2975e-07 0 0]  ProductsOfInertiaUnits=kg*m^2  BasedOnType=Mass  Density=800  DensityUnits=kg/m^3  DoExposeReferenceFrame=on  SerializedFrames=<Frames/>  GraphicType=FromGeometry  MarkerShape=Sphere  MarkerSize=10  GraphicVisPropType=SimpleVisualProperties  GraphicDiffuseColor=[0.5 0.5 0.5]  GraphicSpecularColor=[0.5 0.5 0.5 1.0]  GraphicAmbientColor=[0.15 0.15 0.15 1.0]  GraphicEmissiveColor=[0.0 0.0 0.0 1.0]  GraphicShininess=75  GraphicOpacity=1.0
  PS-Simulink Converter13 : nesl_utility/PS-Simulink Converter  PhysicalDomain=network_engine_domain  SubClassName=ps_output  LeftPortType=input  RightPortType=output  PseudoPeriodic=off  Frequencies=[]  Unit=inherit  AffineConversion=off
      settings: SourceProductBaseCode=PW,SS
  PS-Simulink Converter17 : nesl_utility/PS-Simulink Converter  PhysicalDomain=network_engine_domain  SubClassName=ps_output  LeftPortType=input  RightPortType=output  PseudoPeriodic=off  Frequencies=[]  Unit=inherit  AffineConversion=off
      settings: SourceProductBaseCode=PW,SS
  Spatial Contact Force : sm_lib/Forces and Torques/Spatial Contact Force  CoefficientOfDynamicFriction=0.3  CoefficientOfStaticFriction=0.5  SenseContactBaseRotation=off  SenseContactBaseTranslation=off  NormalDamping=1e3  NormalDampingUnits=N/(m/s)  SenseContactFollowerRotation=off  SenseContactFollowerTranslation=off  SenseContactSignal=off  NormalStiffness=1e6  NormalStiffnessUnits=N/m  FrictionalCriticalVelocity=1e-3  FrictionalCriticalVelocityUnits=m/s  ZeroCrossDetectContactStartAndEnd=off  FrictionType=SmoothStickSlip  SenseFrictionalForceMagnitude=off  SenseNormalForceMagnitude=off  NormalForceType=SmoothSpringDamper  SenseNormalVelocity=off  SenseSeparationDistance=off  SenseTangentialVelocity=off  SenseTangentialVelocityMagnitude=off  NormalTransitionRegionWidth=1e-4  NormalTransitionRegionWidthUnits=m
  Stroke Joint : sm_lib/Joints/Revolute Joint  JointMode=Normal  SenseConstraintForce=off  SenseConstraintForceX=off  SenseConstraintForceY=off  SenseConstraintForceZ=off  SenseConstraintTorque=off  SenseConstraintTorqueX=off  SenseConstraintTorqueY=off  SenseConstraintTorqueZ=off  SenseTotalForce=off  SenseTotalForceX=off  SenseTotalForceY=off  SenseTotalForceZ=off  SenseTotalTorque=off  SenseTotalTorqueX=off  SenseTotalTorqueY=off  SenseTotalTorqueZ=off  CompositeWrenchDir=FollowerOnBase  CompositeWrenchFrame=BaseFrame  EquilibriumPosition=0  EquilibriumPositionUnits=deg  SpringStiffness=stif_stk  SpringStiffnessUnits=N*m/rad  DampingCoefficient=0  DampingCoefficientUnits=N*m/(rad/s)  TorqueActuationMode=ComputedTorque  MotionActuationMode=InputMotion  SensePosition=on  SenseVelocity=on  SenseAcceleration=off  SenseTorqueForce=off  SenseLowerLimitTorqueForce=off  SenseUpperLimitTorqueForce=off  LowerLimitSpecify=on  LowerLimitBound=-90  LowerLimitBoundUnits=deg  LowerLimitStiffness=1e6  LowerLimitStiffnessUnits=N*m/rad  LowerLimitDamping=1e3  LowerLimitDampingUnits=N*m/(rad/s)  LowerLimitTransitionRegionWidth=0.1  LowerLimitTransitionRegionWidthUnits=deg  UpperLimitSpecify=on  UpperLimitBound=90  UpperLimitBoundUnits=deg  UpperLimitStiffness=1e6  UpperLimitStiffnessUnits=N*m/rad  UpperLimitDamping=1e3  UpperLimitDampingUnits=N*m/(rad/s)  UpperLimitTransitionRegionWidth=0.1  UpperLimitTransitionRegionWidthUnits=deg  PositionTargetSpecify=off  PositionTargetPriority=High  PositionTargetValue=-30  PositionTargetValueUnits=deg  VelocityTargetSpecify=off  VelocityTargetPriority=High  VelocityTargetValue=0  VelocityTargetValueUnits=deg/s
  left Shoulder : sm_lib/Frames and Transforms/Rigid Transform  TranslationMethod=Cartesian  TranslationStandardOffset=0  TranslationLengthUnit=cm  TranslationStandardAxis=+Z  TranslationCartesianOffset=[0 1 4]  TranslationROffset=0  TranslationROffsetUnits=m  TranslationZOffset=0  TranslationZOffsetUnits=m  TranslationThetaOffset=0  TranslationThetaOffsetUnits=deg  RotationMethod=StandardAxis  RotationAngleUnits=deg  RotationStandardAxis=+X  RotationAngle=-90  RotationArbitraryAxis=[0 0 1]  FollAlignAxisA=+X  BaseAlignAxisA=+Y  FollAlignAxisB=+Y  BaseAlignAxisB=+Z  RotationSequenceAxes=FollowerAxes  RotationSequence=XYX  RotationSequenceAngles=[0 0 0]  RotationSequenceAnglesUnits=deg  RotationMatrix=[0 1 0; 0 0 1; 1 0 0]
  t of Left Stroke : PMIOPort  Side=Left
  LT : PMIOPort  Port=2  Side=Left
  WT : PMIOPort  Port=3  Side=Right
  G : PMIOPort  Port=4  Side=Right
  Out Bus Element5 : Outport  PortName=left_stk  Element=q
  Out Bus Element6 : Outport  PortName=left_stk  Element=w
  wires:
  PS-Simulink Converter17/1 -> [psi_dot_l]
  PS-Simulink Converter13/1 -> [psi_l]
  [psi_l] -> Out Bus Element5/1
  [psi_dot_l] -> Out Bus Element6/1
  connections:
  Stroke Joint/RConn3 -- PS-Simulink Converter17/LConn1
  Stroke Joint/RConn2 -- PS-Simulink Converter13/LConn1
  Stroke Joint/LConn1 -- LT/RConn1
  Left LE1/RConn1 -- left Shoulder/LConn1 -- Stroke Joint/RConn1
  Stroke Joint/LConn2 -- t of Left Stroke/RConn1
  WT/RConn1 -- left Shoulder/RConn1
  Left LE1/LConn1 -- Spatial Contact Force/RConn1
  Spatial Contact Force/LConn1 -- G/RConn1
